simulink library "env_environment_model_lib"  (R2016b)
settings: Solver=ode45  StartTime=0.0  StopTime=10.0  RelTol=1e-3  EnableMultiTasking=on
values from neighbouring files (symbols this model uses):
  const_gravity_local = single([0, 0,-9.80665])    [env_environment_model_init.m]
  env_ext_air_omega_variance = [0.01 0.01 0.01]    [env_environment_model_init.m]
  env_ext_air_vel_seed = [1 2 3]    [env_environment_model_init.m]
  env_ext_air_vel_variance = [0.01 0.01 0.01]    [env_environment_model_init.m]
  env_grav_disturb_on = boolean(0)    [env_environment_model_init.m]    (also in env_environment_model_test.m)
  env_max_ext_air_omega = single(0.1)    [env_environment_model_init.m]    (also in env_environment_model_test.m)
  env_max_ext_air_vel = single(0.2)    [env_environment_model_init.m]    (also in env_environment_model_test.m)
  env_rotational_drag_coeff = 0.001    [env_environment_model_init.m]
  ini_time_nanoseconds = 0    [env_environment_model_test.m]
  ini_time_seconds = 0    [env_environment_model_test.m]
undefined symbols (not defined in the file or in its folder): astrobee_time_step_size, DiscIntNeverNeededParam, env_avg_drag_coeff, tun_env_accel_dof_gain, tun_env_alpha_dof_gain, tun_env_drag_disturb_on, tun_inertia_error_mat, tun_ini_omega_B_ISS_B, tun_ini_P_B_ISS_ISS, tun_ini_Q_ISS2B, tun_ini_V_B_ISS_ISS, tun_iss_omega_ISS_ECI_ISS, tun_mass_error
libraries: math_utils x8, vrlib x3, simulink x1
settings Model: Creator=jfusco1  LastModifiedBy=jfusco1
settings DataIOCC: LimitDataPoints=on  SaveFormat=Array
settings OptimizationCC: LifeSpan=inf
settings DebuggingCC: SolverPrmCheckMsg=warning  AllowSymbolicDim=off  SFUnexpectedBacktrackingDiag=warning  SFNoUnconditionalDefaultTransitionDiag=warning  SFExecutionAtInitializationDiag=none
settings HardwareCC: ProdBitPerPointer=32  ProdBitPerSizeT=32  ProdBitPerPtrDiffT=32  ProdLargestAtomicFloat=None  ProdIntDivRoundTo=Undefined  ProdEndianess=Unspecified  ProdWordSize=32  ProdHWDeviceType=32-bit Generic
settings ModelReferenceCC: PropagateSignalLabelsOutOfModel=off
settings GRTTargetCC: TargetLangStandard=C89/C90 (ANSI)  GeneratePreprocessorConditionals=Disable all
settings ConfigComp: CovMetricSettings=dw  CovHtmlReporting=on  CovSaveCumulativeToWorkspaceVar=on  CovSaveSingleToWorkspaceVar=on  CovExternalEMLEnable=off  CovSFcnEnable=off

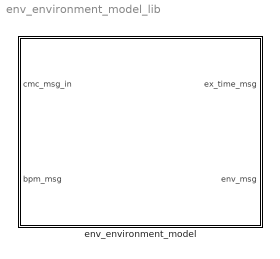
== system env_environment_model_lib ==
  env_environment_model : Subsystem  VariantControl=(default)

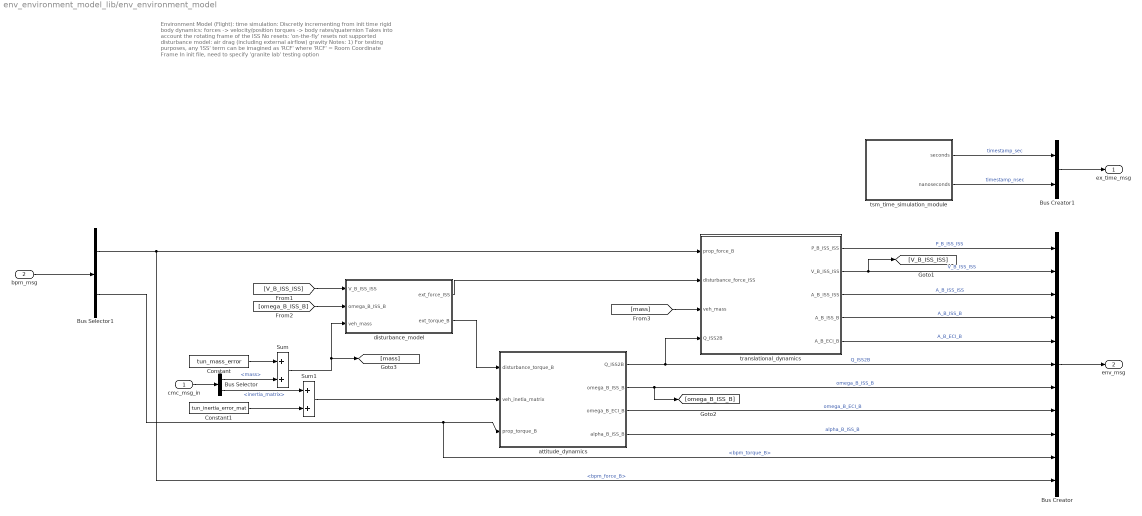
== system env_environment_model_lib/env_environment_model ==
  note: Environment Model (Flight):
      |
      | time simulation:
      | Discretly incrementing from init time
      | rigid body dynamics:
      | forces -> velocity/position
      | torques -> body rates/quaternion
      | Takes into account the rotating frame of the ISS
      | No resets: 'on-the-fly' resets not supported
      | disturbance model:
      | air drag (including external airflow)
      | gravity
      |
      | Notes:
      | 1) For testing purposes, any 'ISS' term can be imagined as 'RCF'
      | where 'RCF' = Room Coordinate Frame
      | In init file, need to specify 'granite lab' testing option
  cmc_msg_in : Inport  OutDataTypeStr=Bus: cmc_msg
  bpm_msg : Inport  Port=2
  Bus Creator : BusCreator  Inputs=11  OutDataTypeStr=Bus: env_msg  NonVirtualBus=on
      settings: InheritFromInputs=off
  Bus Creator1 : BusCreator  Inputs=2  OutDataTypeStr=Bus: ex_time_msg  NonVirtualBus=on
      settings: InheritFromInputs=off
  Bus Selector : BusSelector  OutputSignals=mass,inertia_matrix
  Bus Selector1 : BusSelector  OutputSignals=bpm_force_B,bpm_torque_B
  Constant : Constant  Value=tun_mass_error
  Constant1 : Constant  Value=tun_inertia_error_mat
  Sum : Sum
  Sum1 : Sum
  attitude_dynamics : Subsystem
  disturbance_model : Subsystem
  translational_dynamics : Subsystem
  tsm_time_simulation_module : Subsystem
  ex_time_msg : Outport
  env_msg : Outport  Port=2
  wires:
  bpm_msg/1 -> Bus Selector1/1
  attitude_dynamics/3(omega_B_ECI_B) -> Bus Creator/8  "omega_B_ECI_B"
  [omega_B_ISS_B] -> disturbance_model/2(omega_B_ISS_B)
  translational_dynamics/5(A_B_ECI_B) -> Bus Creator/5  "A_B_ECI_B"
  disturbance_model/2(ext_torque_B) -> attitude_dynamics/1(disturbance_torque_B)
  disturbance_model/1(ext_force_ISS) -> translational_dynamics/2(disturbance_force_ISS)
  [V_B_ISS_ISS] -> disturbance_model/1(V_B_ISS_ISS)
  Bus Creator1/1 -> ex_time_msg/1
  translational_dynamics/1(P_B_ISS_ISS) -> Bus Creator/1  "P_B_ISS_ISS"
  translational_dynamics/2(V_B_ISS_ISS) -> [V_B_ISS_ISS], Bus Creator/2  "V_B_ISS_ISS"
  translational_dynamics/3(A_B_ISS_ISS) -> Bus Creator/3  "A_B_ISS_ISS"
  translational_dynamics/4(A_B_ISS_B) -> Bus Creator/4  "A_B_ISS_B"
  attitude_dynamics/1(Q_ISS2B) -> Bus Creator/6, translational_dynamics/4(Q_ISS2B)  "Q_ISS2B"
  attitude_dynamics/2(omega_B_ISS_B) -> Bus Creator/7, [omega_B_ISS_B]  "omega_B_ISS_B"
  attitude_dynamics/4(alpha_B_ISS_B) -> Bus Creator/9  "alpha_B_ISS_B"
  tsm_time_simulation_module/1(seconds) -> Bus Creator1/1  "timestamp_sec"
  tsm_time_simulation_module/2(nanoseconds) -> Bus Creator1/2  "timestamp_nsec"
  Bus Selector1/1 -> translational_dynamics/1(prop_force_B), Bus Creator/11  "<bpm_force_B>"
  Bus Selector1/2 -> attitude_dynamics/3(prop_torque_B), Bus Creator/10  "<bpm_torque_B>"
  Bus Creator/1 -> env_msg/1
  cmc_msg_in/1 -> Bus Selector/1
  Sum/1 -> disturbance_model/3(veh_mass), [mass]
  [mass] -> translational_dynamics/3(veh_mass)
  Bus Selector/1 -> Sum/2  "<mass>"
  Constant/1 -> Sum/1
  Sum1/1 -> attitude_dynamics/2(veh_inetia_matrix)
  Bus Selector/2 -> Sum1/1  "<inertia_matrix>"
  Constant1/1 -> Sum1/2

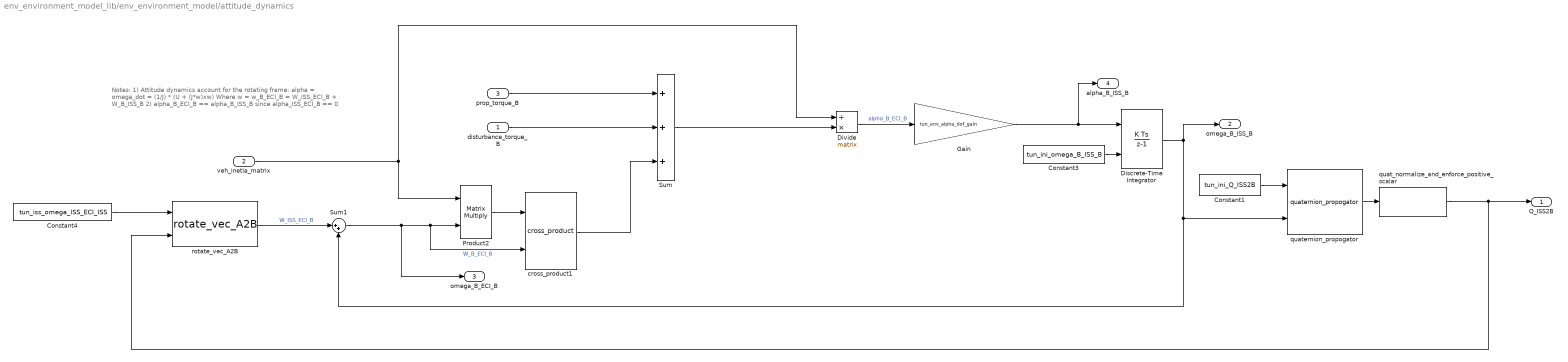
== system env_environment_model_lib/env_environment_model/attitude_dynamics ==
  note: Notes:
      | 	1) Attitude dynamics account for the rotating frame:
      | 		alpha = omega_dot = (1/J) * (U + (J*w)xw)
      | 		Where w = w_B_ECI_B = W_ISS_ECI_B + W_B_ISS_B
      | 	2) alpha_B_ECI_B == alpha_B_ISS_B since alpha_ISS_ECI_B == 0
  disturbance_torque_B : Inport
  veh_inetia_matrix : Inport  Port=2
  prop_torque_B : Inport  Port=3
  Constant1 : Constant  Value=tun_ini_Q_ISS2B
  Constant3 : Constant  Value=tun_ini_omega_B_ISS_B
  Constant4 : Constant  Value=tun_iss_omega_ISS_ECI_ISS
  Discrete-Time Integrator : DiscreteIntegrator  InitialConditionSource=external  InitialConditionSetting=State (most efficient)  SampleTime=astrobee_time_step_size  ICPrevOutput=DiscIntNeverNeededParam  ICPrevScaledInput=DiscIntNeverNeededParam
  Divide : Product  Inputs=/*  Multiplication=Matrix(*)
  Gain : Gain  Gain=tun_env_alpha_dof_gain
  Product2 : Product  Multiplication=Matrix(*)
  Sum : Sum  Inputs=+++
  Sum1 : Sum  Inputs=|++
  cross_product1 : math_utils/cross_product  SystemSampleTime=-1
  quat_normalize_and_enforce_positive_scalar : math_utils/quat_normalize_and_enforce_positive_scalar  SystemSampleTime=-1
  quaternion_propogator : math_utils/quaternion_propogator
  rotate_vec_A2B : math_utils/rotate_vec_A2B  SystemSampleTime=-1
  Q_ISS2B : Outport
  omega_B_ISS_B : Outport  Port=2
  omega_B_ECI_B : Outport  Port=3
  alpha_B_ISS_B : Outport  Port=4
  wires:
  Discrete-Time Integrator/1 -> Sum1/2, quaternion_propogator/2, omega_B_ISS_B/1
  Constant1/1 -> quaternion_propogator/1
  quat_normalize_and_enforce_positive_scalar/1 -> rotate_vec_A2B/2, Q_ISS2B/1
  veh_inetia_matrix/1 -> Product2/1, Divide/1
  Divide/1 -> Gain/1  "alpha_B_ECI_B"
  prop_torque_B/1 -> Sum/1
  cross_product1/1 -> Sum/3
  Sum/1 -> Divide/2
  Product2/1 -> cross_product1/1
  Constant3/1 -> Discrete-Time Integrator/2
  Sum1/1 -> omega_B_ECI_B/1, cross_product1/2, Product2/2  "W_B_ECI_B"
  rotate_vec_A2B/1 -> Sum1/1  "W_ISS_ECI_B"
  Constant4/1 -> rotate_vec_A2B/1
  disturbance_torque_B/1 -> Sum/2
  Gain/1 -> alpha_B_ISS_B/1, Discrete-Time Integrator/1
  quaternion_propogator/1 -> quat_normalize_and_enforce_positive_scalar/1

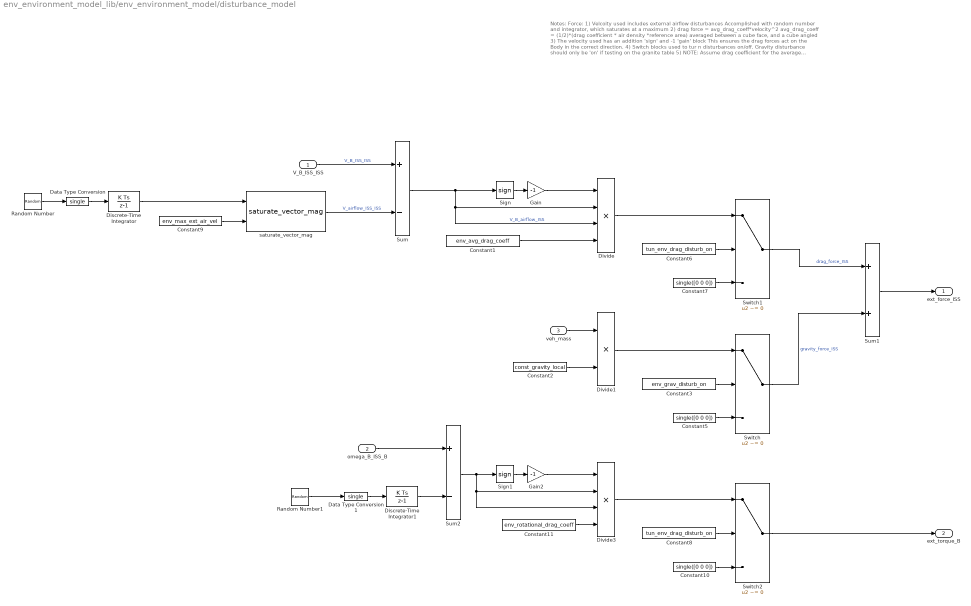
== system env_environment_model_lib/env_environment_model/disturbance_model ==
  note: Notes:
      |
      | Force:
      | 	1) Velcoity used includes external airflow disturbances
      | 		Accomplished with random number and integrator, which saturates  at a maximum
      | 	2) drag force = avg_drag_coeff*velocity^2
      | 		avg_drag_coeff = (1/2)*(drag coefficient * air density *reference area)
      | 			averaged between a cube face, and a cube angled
      | 	3) The velocity used has an addition 'sign' and -1 'gain' block
      | 		This ensures the drag forces act on the Body in the correct direction.
      | 	4) Switch blocks used to tur n disturbances on/off.
      | 		Gravity disturbance should only be 'on' if testing on the granite table
      | 	5) NOTE: Assume drag coefficient for the average between a cube face and cube angle.
      | 		Fairly similar values for each, so average to remove need to account for orientation
      |
      | Torque:
      | 	1) No direct model could be found to relate a rotating cube to drag
      | 	2) Simply uses a factor value (in conjunction with the -1) to create some relative force in the opposite direction
  V_B_ISS_ISS : Inport
  omega_B_ISS_B : Inport  Port=2
  veh_mass : Inport  Port=3
  Constant1 : Constant  Value=env_avg_drag_coeff
  Constant10 : Constant  Value=single([0 0 0])
  Constant11 : Constant  Value=env_rotational_drag_coeff
  Constant2 : Constant  Value=const_gravity_local
  Constant3 : Constant  Value=env_grav_disturb_on
  Constant5 : Constant  Value=single([0 0 0])
  Constant6 : Constant  Value=tun_env_drag_disturb_on
  Constant7 : Constant  Value=single([0 0 0])
  Constant8 : Constant  Value=tun_env_drag_disturb_on
  Constant9 : Constant  Value=env_max_ext_air_vel
  Data Type Conversion : DataTypeConversion  OutDataTypeStr=single
  Data Type Conversion1 : DataTypeConversion  OutDataTypeStr=single
  Discrete-Time Integrator : DiscreteIntegrator  InitialConditionSetting=State (most efficient)  SampleTime=-1  LimitOutput=on  UpperSaturationLimit=env_max_ext_air_vel  LowerSaturationLimit=-(env_max_ext_air_vel+eps)  ICPrevOutput=DiscIntNeverNeededParam  ICPrevScaledInput=DiscIntNeverNeededParam
      settings: AttributesFormatString=|
      | IC:%<InitialCondition>
      | sat limit: %<UpperSaturationLimit>
  Discrete-Time Integrator1 : DiscreteIntegrator  InitialConditionSetting=State (most efficient)  SampleTime=-1  LimitOutput=on  UpperSaturationLimit=env_max_ext_air_omega  LowerSaturationLimit=-(env_max_ext_air_omega+eps)  ICPrevOutput=DiscIntNeverNeededParam  ICPrevScaledInput=DiscIntNeverNeededParam
      settings: AttributesFormatString=|
      | IC:%<InitialCondition>
      | sat limit: %<UpperSaturationLimit>
  Divide : Product  Inputs=****
  Divide1 : Product  Inputs=**
  Divide3 : Product  Inputs=****
  Gain : Gain  Gain=-1
  Gain2 : Gain  Gain=-1
  Random Number : RandomNumber  Variance=env_ext_air_vel_variance  Seed=env_ext_air_vel_seed  SampleTime=astrobee_time_step_size
      settings: AttributesFormatString=|
      | Mean: %<Mean>
      | Variance: %<Variance>
      | Seed: %<Seed>
      | SampleTime: %<SampleTime>
  Random Number1 : RandomNumber  Variance=env_ext_air_omega_variance  Seed=env_ext_air_vel_seed  SampleTime=astrobee_time_step_size
      settings: AttributesFormatString=|
      | Mean: %<Mean>
      | Variance: %<Variance>
      | Seed: %<Seed>
      | SampleTime: %<SampleTime>
  Sign : Signum
  Sign1 : Signum
  Sum : Sum  Inputs=+-
  Sum1 : Sum
  Sum2 : Sum  Inputs=+-
  Switch : Switch  Criteria=u2 ~= 0
  Switch1 : Switch  Criteria=u2 ~= 0
  Switch2 : Switch  Criteria=u2 ~= 0
  saturate_vector_mag : math_utils/saturate_vector_mag  SystemSampleTime=-1
  ext_force_ISS : Outport
  ext_torque_B : Outport  Port=2
  wires:
  Sum2/1 -> Sign1/1, Divide3/2, Divide3/3
  Divide3/1 -> Switch2/1
  Gain2/1 -> Divide3/1
  Sign1/1 -> Gain2/1
  Discrete-Time Integrator1/1 -> Sum2/2
  Random Number1/1 -> Data Type Conversion1/1
  Data Type Conversion1/1 -> Discrete-Time Integrator1/1
  omega_B_ISS_B/1 -> Sum2/1
  Constant11/1 -> Divide3/4
  Switch2/1 -> ext_torque_B/1
  Constant10/1 -> Switch2/3
  Constant8/1 -> Switch2/2
  Gain/1 -> Divide/1
  Sign/1 -> Gain/1
  Constant9/1 -> saturate_vector_mag/2
  Discrete-Time Integrator/1 -> saturate_vector_mag/1
  Data Type Conversion/1 -> Discrete-Time Integrator/1
  Divide/1 -> Switch1/1
  Constant7/1 -> Switch1/3
  Constant6/1 -> Switch1/2
  Constant5/1 -> Switch/3
  Constant3/1 -> Switch/2
  Switch/1 -> Sum1/2  "gravity_force_ISS"
  V_B_ISS_ISS/1 -> Sum/1  "V_B_ISS_ISS"
  Divide1/1 -> Switch/1
  Constant2/1 -> Divide1/2
  veh_mass/1 -> Divide1/1
  Sum1/1 -> ext_force_ISS/1
  Switch1/1 -> Sum1/1  "drag_force_ISS"
  saturate_vector_mag/1 -> Sum/2  "V_airflow_ISS_ISS"
  Sum/1 -> Divide/2, Divide/3, Sign/1  "V_B_airflow_ISS"
  Random Number/1 -> Data Type Conversion/1
  Constant1/1 -> Divide/4

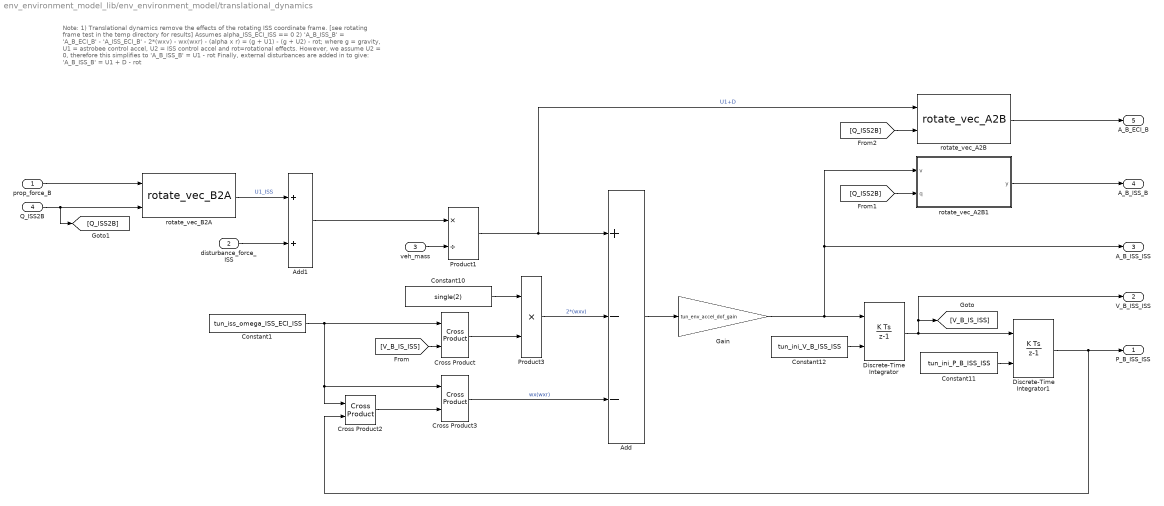
== system env_environment_model_lib/env_environment_model/translational_dynamics ==
  note: Note:
      | 	1) Translational dynamics remove the effects of the rotating ISS coordinate frame.  [see rotating frame test in the temp directory for results]
      | 		Assumes alpha_ISS_ECI_ISS == 0
      | 	2) 'A_B_ISS_B' = 'A_B_ECI_B' - 'A_ISS_ECI_B' -  2*(wxv) - wx(wxr) - (alpha x r)
      | 			= (g + U1) - (g + U2) - rot; where g = gravity, U1 = astrobee control accel, U2 = ISS control accel and rot=rotational effects.
      | 		However, we assume U2 = 0, therefore this simplifies to 'A_B_ISS_B' = U1 - rot
      | 		Finally, external disturbances are added in to give: 'A_B_ISS_B' = U1 + D - rot
  prop_force_B : Inport
  disturbance_force_ISS : Inport  Port=2
  veh_mass : Inport  Port=3
  Q_ISS2B : Inport  Port=4
  Add : Sum  Inputs=+--
  Add1 : Sum
  Constant1 : Constant  Value=tun_iss_omega_ISS_ECI_ISS
  Constant10 : Constant  Value=single(2)
  Constant11 : Constant  Value=tun_ini_P_B_ISS_ISS
  Constant12 : Constant  Value=tun_ini_V_B_ISS_ISS
  Cross Product : vrlib/Utilities/Cross Product
  Cross Product2 : vrlib/Utilities/Cross Product
  Cross Product3 : vrlib/Utilities/Cross Product
  Discrete-Time Integrator : DiscreteIntegrator  InitialConditionSource=external  InitialConditionSetting=State (most efficient)  SampleTime=astrobee_time_step_size  ICPrevOutput=DiscIntNeverNeededParam  ICPrevScaledInput=DiscIntNeverNeededParam
  Discrete-Time Integrator1 : DiscreteIntegrator  InitialConditionSource=external  InitialConditionSetting=State (most efficient)  SampleTime=astrobee_time_step_size  ICPrevOutput=DiscIntNeverNeededParam  ICPrevScaledInput=DiscIntNeverNeededParam
  Gain : Gain  Gain=tun_env_accel_dof_gain
  Product1 : Product  Inputs=*/
  Product3 : Product
  rotate_vec_A2B : math_utils/rotate_vec_A2B  SystemSampleTime=-1
  rotate_vec_A2B1 : Subsystem
      mask Display:
      | disp('Rotate Vector\n\n')
      | disp('A to B');
  rotate_vec_B2A : math_utils/rotate_vec_B2A  SystemSampleTime=-1
  P_B_ISS_ISS : Outport
  V_B_ISS_ISS : Outport  Port=2
  A_B_ISS_ISS : Outport  Port=3
  A_B_ISS_B : Outport  Port=4
  A_B_ECI_B : Outport  Port=5
  wires:
  [Q_ISS2B] -> rotate_vec_A2B/2
  rotate_vec_A2B/1 -> A_B_ECI_B/1
  Discrete-Time Integrator/1 -> V_B_ISS_ISS/1, [V_B_IS_ISS], Discrete-Time Integrator1/1
  Constant1/1 -> Cross Product3/1, Cross Product2/1, Cross Product/1
  Discrete-Time Integrator1/1 -> P_B_ISS_ISS/1, Cross Product2/2
  Cross Product2/1 -> Cross Product3/2
  Constant10/1 -> Product3/1
  Cross Product/1 -> Product3/2
  Product3/1 -> Add/2  "2*(wxv)"
  Constant12/1 -> Discrete-Time Integrator/2
  Constant11/1 -> Discrete-Time Integrator1/2
  Add/1 -> Gain/1
  Cross Product3/1 -> Add/3  "wx(wxr)"
  Product1/1 -> rotate_vec_A2B/1, Add/1  "U1+D"
  prop_force_B/1 -> rotate_vec_B2A/1
  Q_ISS2B/1 -> rotate_vec_B2A/2, [Q_ISS2B]
  [V_B_IS_ISS] -> Cross Product/2
  rotate_vec_A2B1/1(y) -> A_B_ISS_B/1
  [Q_ISS2B] -> rotate_vec_A2B1/2(q)
  veh_mass/1 -> Product1/2
  Add1/1 -> Product1/1
  rotate_vec_B2A/1 -> Add1/1  "U1_ISS"
  disturbance_force_ISS/1 -> Add1/2
  Gain/1 -> Discrete-Time Integrator/1, rotate_vec_A2B1/1(v), A_B_ISS_ISS/1

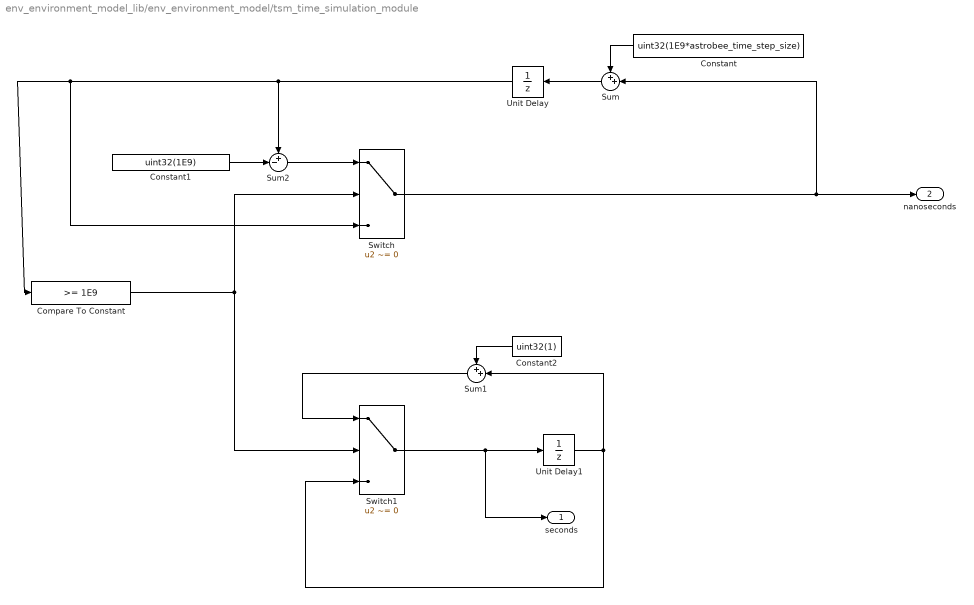
== system env_environment_model_lib/env_environment_model/tsm_time_simulation_module ==
  Compare To Constant : simulink/Logic and Bit Operations/Compare To Constant  relop=>=  const=1E9  OutDataTypeStr=boolean
  Constant : Constant  Value=uint32(1E9*astrobee_time_step_size)
  Constant1 : Constant  Value=uint32(1E9)
  Constant2 : Constant  Value=uint32(1)
  Sum : Sum  Inputs=++|
  Sum1 : Sum  Inputs=++|
  Sum2 : Sum  Inputs=+-|
  Switch : Switch  Criteria=u2 ~= 0
  Switch1 : Switch  Criteria=u2 ~= 0
  Unit Delay : UnitDelay  InitialCondition=ini_time_nanoseconds  SampleTime=-1
      settings: AttributesFormatString=IC: %<InitialCondition>
  Unit Delay1 : UnitDelay  InitialCondition=ini_time_seconds  SampleTime=-1
      settings: AttributesFormatString=IC: %<InitialCondition>
  seconds : Outport
  nanoseconds : Outport  Port=2
  wires:
  Constant1/1 -> Sum2/2
  Switch/1 -> nanoseconds/1, Sum/2
  Unit Delay/1 -> Sum2/1, Compare To Constant/1, Switch/3
  Sum/1 -> Unit Delay/1
  Sum1/1 -> Switch1/1
  Constant2/1 -> Sum1/1
  Switch1/1 -> Unit Delay1/1, seconds/1
  Unit Delay1/1 -> Switch1/3, Sum1/2
  Sum2/1 -> Switch/1
  Compare To Constant/1 -> Switch1/2, Switch/2
  Constant/1 -> Sum/1

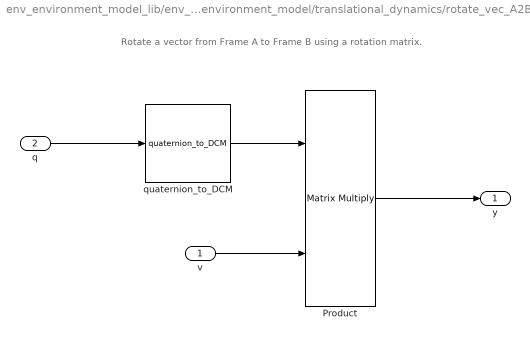
== system env_environment_model_lib/env_environment_model/translational_dynamics/rotate_vec_A2B1 ==
  note: Rotate a vector from Frame A to Frame B using a rotation matrix.
  v : Inport
  q : Inport  Port=2  PortDimensions=4
  Product : Product  Multiplication=Matrix(*)
  quaternion_to_DCM : math_utils/quaternion_to_DCM  SystemSampleTime=-1
  y : Outport
  wires:
  Product/1 -> y/1
  v/1 -> Product/2
  quaternion_to_DCM/1 -> Product/1
  q/1 -> quaternion_to_DCM/1
